simulink model "untitled"  (R2023b)
settings: Solver=VariableStepAuto  StartTime=0.0  StopTime=10.0  RelTol=1e-3
values from neighbouring files (symbols this model uses):
  A = [0 1;-(kf)/(m) -(cf)/(m)]    [Lab6_damping.m]    (also in editer.m = zeros(1000,1); fortnite.m = [; fortniteV2.m = [; fortnite_DampPlot.m = [)
  B = randi([1,100])/100    [fitter.m]    (also in fortnite.m = [; fortniteV2.m = [; fortnite_DampPlot.m = [)
  C = randi([-15000,100])/10000    [fitter.m]    (also in fortniteV2.m = [1 0 0 0 0 0 0 0 0 0 0 0 0 0)
  D = randi([round(1000*(ymax-ymax*.2)),round(1000*(ymax+ymax*.2))])/1000    [fitter.m]    (also in fortniteV2.m = zeros(14,4))
settings Model: Creator=elija  LastModifiedBy=elija

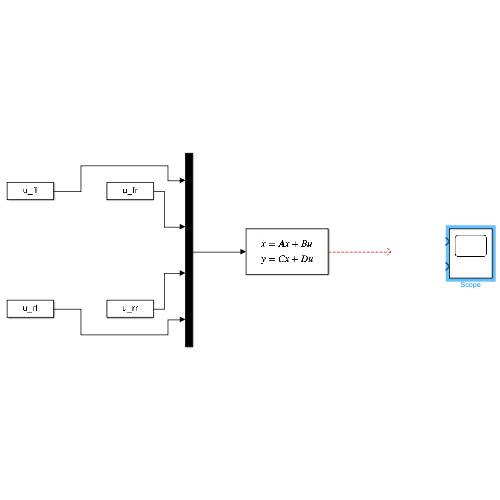
[thumbnail: Simulink's stored preview of the top-level diagram]
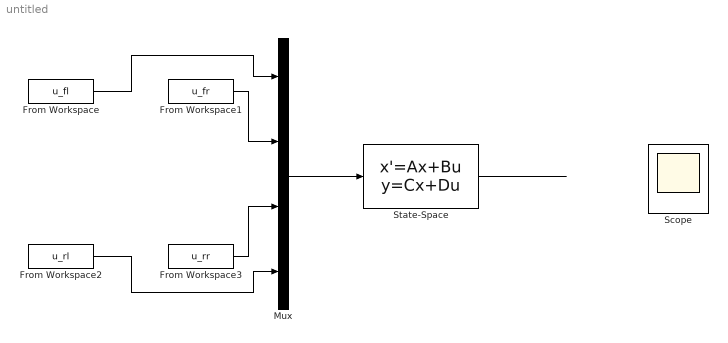
== system untitled ==
  From Workspace : FromWorkspace  VariableName=u_fl
  From Workspace1 : FromWorkspace  VariableName=u_fr
  From Workspace2 : FromWorkspace  VariableName=u_rl
  From Workspace3 : FromWorkspace  VariableName=u_rr
  Mux : Mux
  Scope : Scope  NumInputPorts=2
  State-Space : StateSpace  A=A  B=B  C=C  D=D  InitialCondition=0
  wires:
  From Workspace/1 -> Mux/1
  From Workspace1/1 -> Mux/2
  From Workspace2/1 -> Mux/4
  From Workspace3/1 -> Mux/3
  Mux/1 -> State-Space/1
  State-Space/1 -> ?
